simulink model "Sliding_mode"  (R2020a)
settings: Solver=FixedStepAuto  StartTime=0.0  StopTime=20  FixedStep=Ts  RelTol=1e-3
values from neighbouring files (symbols this model uses):
  K1 = 5*g/7    (= 7.00714285714)    [Sliding_mode.m]
  lambda = 2    [Sliding_mode.m]
  Ts = 0.02    [Sliding_mode.m]
undefined symbols (not defined in the file or in its folder): K
libraries: simulink x3
settings Model: Creator=Ashraf  LastModifiedBy=hhiastt
settings DataIOCC: ReturnWorkspaceOutputs=off
settings DebuggingCC: ArithmeticOperatorsInVariantConditions=warning
settings SFSimCC: SimUseLocalCustomCode=off  CustomCodeUndefinedFunction=UseInterfaceOnly
settings RTWCC: RTWUseLocalCustomCode=off
settings CodeAppCC: StateflowObjectComments=on

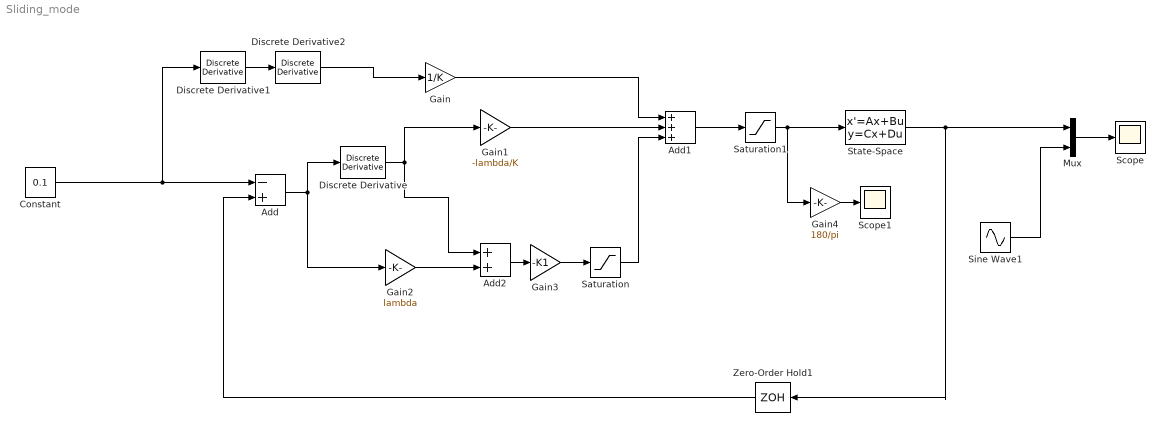
== system Sliding_mode ==
  Add : Sum  Inputs=-+
  Add1 : Sum  Inputs=+++
  Add2 : Sum
  Constant : Constant  Value=0.1
  Discrete Derivative : simulink/Discrete/Discrete Derivative  gainval=1.0  ICPrevScaledInput=0.0  OutMin=[]  OutMax=[]  OutDataType=fixdt(1, 16)  OutScaling=2^-10  DoSatur=off
  Discrete Derivative1 : simulink/Discrete/Discrete Derivative  gainval=1.0  ICPrevScaledInput=0.0  OutMin=[]  OutMax=[]  OutDataType=fixdt(1, 16)  OutScaling=2^-10  DoSatur=off
  Discrete Derivative2 : simulink/Discrete/Discrete Derivative  gainval=1.0  ICPrevScaledInput=0.0  OutMin=[]  OutMax=[]  OutDataType=fixdt(1, 16)  OutScaling=2^-10  DoSatur=off
  Gain : Gain  Gain=1/K
  Gain1 : Gain  Gain=-lambda/K
  Gain2 : Gain  Gain=lambda
  Gain3 : Gain  Gain=-K1
  Gain4 : Gain  Gain=180/pi
  Mux : Mux  Inputs=2
  Saturation : Saturate  ZeroCross=off
  Saturation1 : Saturate  UpperLimit=5*pi/180  LowerLimit=-5*pi/180  ZeroCross=off
  Scope : Scope
  Scope1 : Scope
  Sine Wave1 : Sin  Amplitude=0.2  Frequency=0.25  SampleTime=0
  State-Space : StateSpace  A=[0 1;0 0]  B=[0;K]  C=[1 0]  D=0  InitialCondition=[0 0]
  Zero-Order Hold1 : ZeroOrderHold  SampleTime=Ts
  wires:
  Discrete Derivative2/1 -> Gain/1
  Add/1 -> Discrete Derivative/1, Gain2/1
  Gain/1 -> Add1/1
  Gain1/1 -> Add1/2
  Discrete Derivative/1 -> Add2/1, Gain1/1
  Gain3/1 -> Saturation/1
  Add2/1 -> Gain3/1
  Saturation/1 -> Add1/3
  Gain2/1 -> Add2/2
  Add1/1 -> Saturation1/1
  State-Space/1 -> Zero-Order Hold1/1, Mux/1
  Gain4/1 -> Scope1/1
  Constant/1 -> Add/1, Discrete Derivative1/1
  Sine Wave1/1 -> Mux/2
  Mux/1 -> Scope/1
  Discrete Derivative1/1 -> Discrete Derivative2/1
  Saturation1/1 -> State-Space/1, Gain4/1
  Zero-Order Hold1/1 -> Add/2
